simulink model "s_2012"  (Simulink 7.9)
settings: Solver=ode3  SolverMode=SingleTasking  StartTime=0.0  StopTime=10  FixedStep=0.02  MaxStep=0.02  MinStep=0.02  RelTol=1e-3
model workspace: external: MATLAB File I:\mat\ADRC\ass.m (data not in the file)
values from neighbouring files (symbols this model uses):
  a0 = 0.5    [ass.m]    (also in fcn.m = (d^2+8*r*abs(y))^0.5)
  a1 = 0.4    [ass.m]
  a2 = 0.75    [ass.m]
  delta0 = 0.001    [ass.m]
  delta1 = 0.001    [ass.m]
  delta2 = 0.001    [ass.m]
undefined symbols (not defined in the file or in its folder): DiscIntNeverNeededParam
settings Model: Creator=Administrator  LastModifiedBy=Administrator  CovMetricSettings=dwe  CovHtmlReporting=off  covSaveCumulativeToWorkspaceVar=off  CovSaveSingleToWorkspaceVar=off  CovExternalEMLEnable=on
settings SolverCC: InitialStep=0.02
settings DataIOCC: LimitDataPoints=off  SaveFormat=StructureWithTime  SignalLoggingSaveFormat=Dataset  ReturnWorkspaceOutputs=on
settings OptimizationCC: ExpressionDepthLimit=128
settings DebuggingCC: UnderspecifiedInitializationDetection=Simplified  MergeDetectMultiDrivingBlocksExec=error  SolverPrmCheckMsg=none  FrameProcessingCompatibilityMsg=error  StateNameClashWarn=none  SFUnexpectedBacktrackingDiag=error  SFNoUnconditionalDefaultTransitionDiag=error
settings HardwareCC: ProdBitPerPointer=64  ProdLargestAtomicFloat=Float  ProdIntDivRoundTo=Zero  ProdEndianess=LittleEndian  ProdHWDeviceType=Specified
settings ModelReferenceCC: PropagateSignalLabelsOutOfModel=on
settings SFSimCC: SimUseLocalCustomCode=on
settings RTWCC: RTWUseLocalCustomCode=on
settings CodeAppCC: CustomSymbolStrType=$N$R$M_T
settings GRTTargetCC: CodeReplacementLibrary=C99 (ISO)  GeneratePreprocessorConditionals=Use local settings

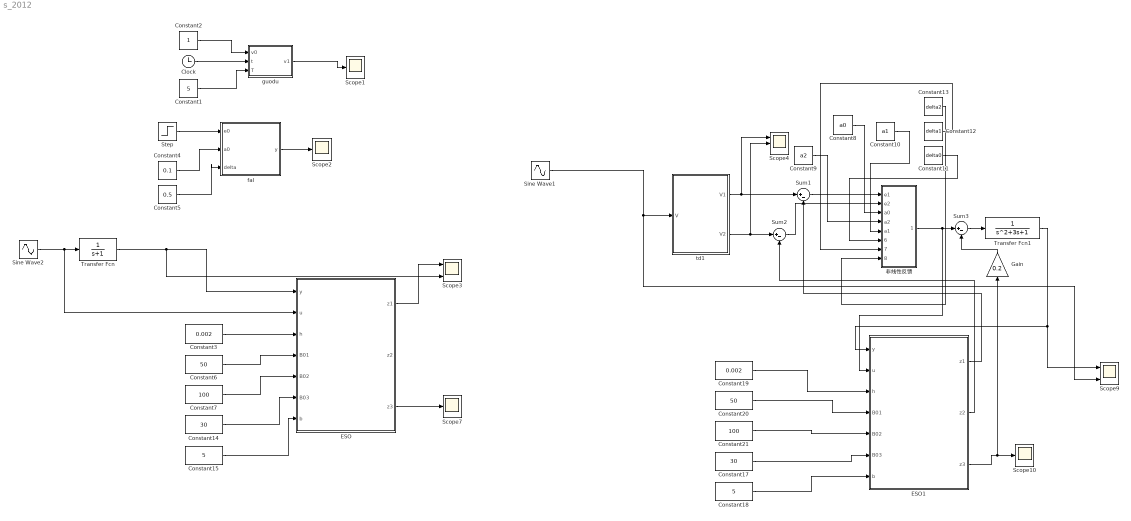
== system s_2012 ==
  Clock : Clock
  Constant1 : Constant  Value=5
  Constant10 : Constant  Value=a1
  Constant11 : Constant  Value=delta0
  Constant12 : Constant  Value=delta1
  Constant13 : Constant  Value=delta2
  Constant14 : Constant  Value=30
  Constant15 : Constant  Value=5
  Constant17 : Constant  Value=30
  Constant18 : Constant  Value=5
  Constant19 : Constant  Value=0.002
  Constant2 : Constant
  Constant20 : Constant  Value=50
  Constant21 : Constant  Value=100
  Constant3 : Constant  Value=0.002
  Constant4 : Constant  Value=0.1
  Constant5 : Constant  Value=0.5
  Constant6 : Constant  Value=50
  Constant7 : Constant  Value=100
  Constant8 : Constant  Value=a0
  Constant9 : Constant  Value=a2
  ESO : Subsystem
  ESO1 : Subsystem
  Gain : Gain  Gain=0.2
  Scope{1..2,7,10} (4 alike) : Scope
      Scope1 settings: TimeRange=auto  MaxDataPoints=5000  SaveToWorkspace=off  YMin=-0.125  YMax=1.125  SampleTime=-1
      Scope10 settings: TimeRange=auto  MaxDataPoints=5000  SaveToWorkspace=off  SaveName=ScopeData3  YMin=-6.92252  YMax=6.95171  SampleTime=-1
      Scope2 settings: TimeRange=auto  MaxDataPoints=5000  SaveToWorkspace=off  SaveName=ScopeData2  YMin=-0.125  YMax=1.125  SampleTime=-1
      Scope7 settings: TimeRange=auto  MaxDataPoints=5000  SaveToWorkspace=off  SaveName=ScopeData8  YMin=-6.95031  YMax=6.9548  SampleTime=-1
  Scope3 : Scope  NumInputPorts=2
      settings: TimeRange=auto  MaxDataPoints=5000  SaveToWorkspace=off  YMin=-0.89002~-5  YMax=0.93911~5  SampleTime=-1
  Scope4 : Scope  NumInputPorts=3
      settings: TimeRange=auto  MaxDataPoints=5000  SaveToWorkspace=off  SaveName=ScopeData3  YMin=-3.68521~-5~-5  YMax=4.43656~5~5  SampleTime=-1
  Scope9 : Scope  NumInputPorts=2
      settings: TimeRange=auto  MaxDataPoints=5000  SaveToWorkspace=off  SaveName=ScopeData4  YMin=-1.45701~-5  YMax=1.50602~5  SampleTime=-1
  Sine Wave1 : Sin  SampleTime=0
  Sine Wave2 : Sin  SampleTime=0
  Step : Step  SampleTime=0
  Sum1 : Sum  Inputs=|+-
  Sum2 : Sum  Inputs=|+-
  Sum3 : Sum  Inputs=|+-
  Transfer Fcn : TransferFcn  Denominator=[1 1]
  Transfer Fcn1 : TransferFcn  Denominator=[1 3 1]
  fal : MATLAB Function  TreatAsAtomicUnit=on
      settings: PermitHierarchicalResolution=ParametersOnly
  guodu : MATLAB Function  TreatAsAtomicUnit=on
      settings: PermitHierarchicalResolution=ParametersOnly
  td1 : Subsystem
  非线性反馈 : Subsystem
  wires:
  Clock/1 -> guodu/2(t)
  Constant1/1 -> guodu/3(T)
  Constant2/1 -> guodu/1(v0)
  guodu/1(v1) -> Scope1/1
  Step/1 -> fal/1(e0)
  Constant4/1 -> fal/2(a0)
  Constant5/1 -> fal/3(delta)
  fal/1(y) -> Scope2/1
  td1/1(V1) -> Scope4/1, Sum1/1
  Sum1/1 -> 非线性反馈/1(e1)
  td1/2(V2) -> Scope4/2, Sum2/1
  Sum2/1 -> 非线性反馈/2(e2)
  Constant10/1 -> 非线性反馈/5(a1)
  Constant9/1 -> 非线性反馈/4(a2)
  Constant8/1 -> 非线性反馈/3(a0)
  Constant11/1 -> 非线性反馈/6(delta0)
  Constant12/1 -> 非线性反馈/7(delta1)
  Constant13/1 -> 非线性反馈/8(delta2)
  Constant3/1 -> ESO/3(h)
  Constant6/1 -> ESO/4(B01)
  Constant7/1 -> ESO/5(B02)
  Constant14/1 -> ESO/6(B03)
  Constant15/1 -> ESO/7(b)
  ESO1/2(z2) -> Sum2/2
  ESO/3(z3) -> Scope7/1
  Sine Wave2/1 -> ESO/2(u), Transfer Fcn/1
  Transfer Fcn/1 -> Scope3/2, ESO/1(y)
  ESO/1(z1) -> Scope3/1
  ESO1/3(z3) -> Gain/1, Scope10/1
  Constant18/1 -> ESO1/7(b)
  Constant17/1 -> ESO1/6(B03)
  Constant21/1 -> ESO1/5(B02)
  Constant19/1 -> ESO1/3(h)
  Constant20/1 -> ESO1/4(B01)
  非线性反馈/1(Out1) -> Sum3/1, ESO1/2(u)
  ESO1/1(z1) -> Sum1/2
  Transfer Fcn1/1 -> ESO1/1(y), Scope9/1
  Sine Wave1/1 -> Scope9/2, td1/1(V)
  Sum3/1 -> Transfer Fcn1/1
  Gain/1 -> Sum3/2

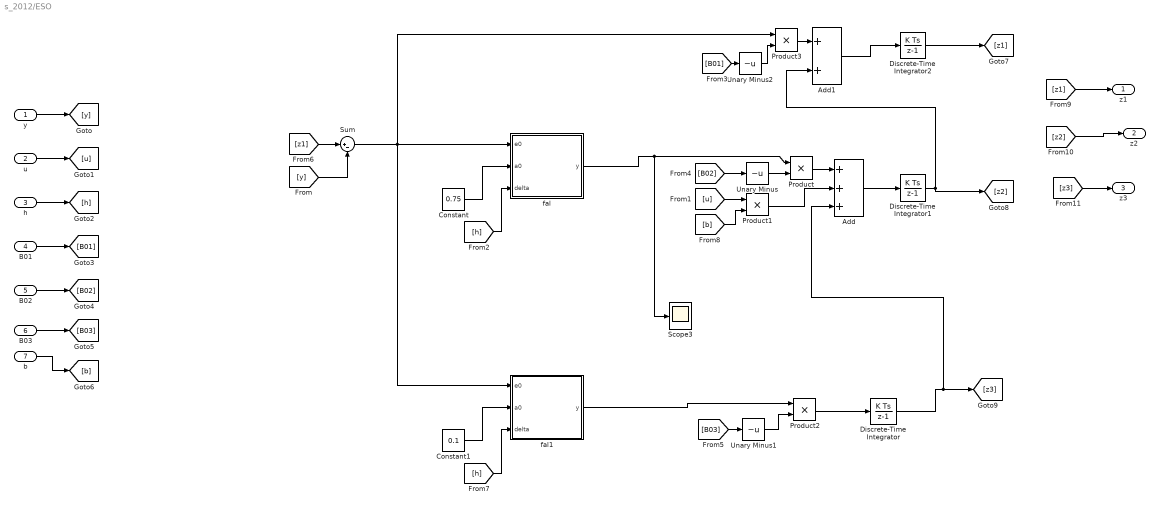
== system s_2012/ESO ==
  y : Inport
  u : Inport  Port=2
  h : Inport  Port=3
  B01 : Inport  Port=4
  B02 : Inport  Port=5
  B03 : Inport  Port=6
  b : Inport  Port=7
  Add : Sum  Inputs=+++
  Add1 : Sum
  Constant : Constant  Value=0.75
  Constant1 : Constant  Value=0.1
  Discrete-Time Integrator : DiscreteIntegrator  InitialConditionMode=State only (most efficient)  SampleTime=-1  ICPrevOutput=DiscIntNeverNeededParam  ICPrevScaledInput=DiscIntNeverNeededParam
  Discrete-Time Integrator1 : DiscreteIntegrator  InitialConditionMode=State only (most efficient)  SampleTime=-1  ICPrevOutput=DiscIntNeverNeededParam  ICPrevScaledInput=DiscIntNeverNeededParam
  Discrete-Time Integrator2 : DiscreteIntegrator  InitialConditionMode=State only (most efficient)  SampleTime=-1  ICPrevOutput=DiscIntNeverNeededParam  ICPrevScaledInput=DiscIntNeverNeededParam
  Product{,1..3} (4 alike) : Product
  Scope3 : Scope
      settings: TimeRange=auto  MaxDataPoints=5000  SaveToWorkspace=off  SaveName=ScopeData2  YMin=-0.00703  YMax=0.01145  SampleTime=-1
  Sum : Sum  Inputs=|+-
  Unary Minus : UnaryMinus
  Unary Minus1 : UnaryMinus
  Unary Minus2 : UnaryMinus
  fal : MATLAB Function  TreatAsAtomicUnit=on
      settings: PermitHierarchicalResolution=ParametersOnly
  fal1 : MATLAB Function  TreatAsAtomicUnit=on
      settings: PermitHierarchicalResolution=ParametersOnly
  z1 : Outport
  z2 : Outport  Port=2
  z3 : Outport  Port=3
  wires:
  y/1 -> [y]
  u/1 -> [u]
  h/1 -> [h]
  B01/1 -> [B01]
  B02/1 -> [B02]
  B03/1 -> [B03]
  [h] -> fal/3(delta)
  [z1] -> Sum/1
  [y] -> Sum/2
  Constant/1 -> fal/2(a0)
  Constant1/1 -> fal1/2(a0)
  [h] -> fal1/3(delta)
  b/1 -> [b]
  [B02] -> Unary Minus/1
  Unary Minus/1 -> Product/2
  [u] -> Product1/1
  [b] -> Product1/2
  Product1/1 -> Add/2
  Product/1 -> Add/1
  fal/1(y) -> Scope3/1, Product/1
  [B03] -> Unary Minus1/1
  Unary Minus1/1 -> Product2/2
  fal1/1(y) -> Product2/1
  [B01] -> Unary Minus2/1
  Sum/1 -> Product3/1, fal1/1(e0), fal/1(e0)
  Unary Minus2/1 -> Product3/2
  Product2/1 -> Discrete-Time Integrator/1
  Add/1 -> Discrete-Time Integrator1/1
  Discrete-Time Integrator2/1 -> [z1]
  Discrete-Time Integrator1/1 -> Add1/2, [z2]
  Discrete-Time Integrator/1 -> Add/3, [z3]
  Product3/1 -> Add1/1
  Add1/1 -> Discrete-Time Integrator2/1
  [z1] -> z1/1
  [z2] -> z2/1
  [z3] -> z3/1

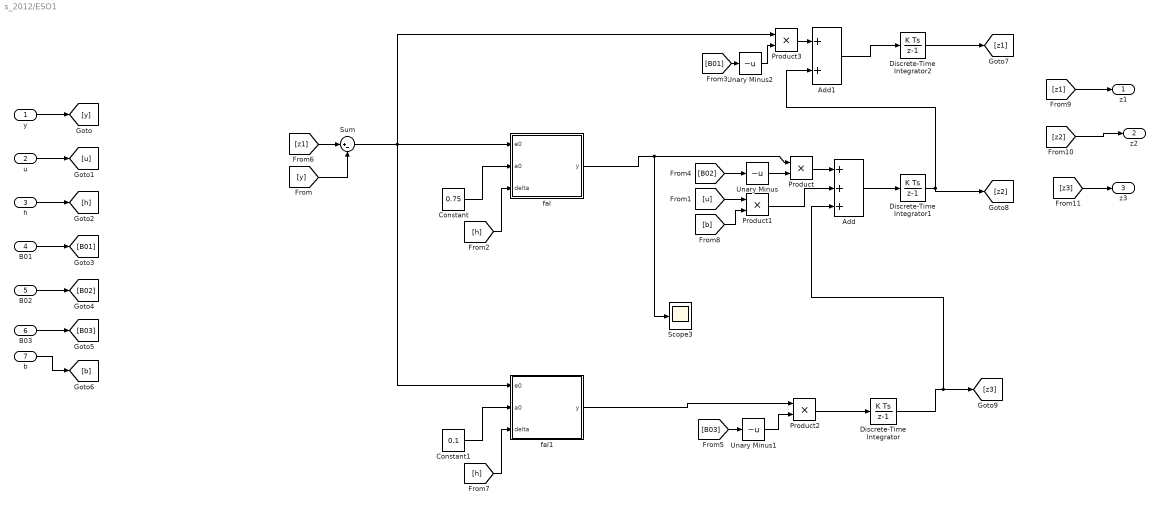
== system s_2012/ESO1 ==
  y : Inport
  u : Inport  Port=2
  h : Inport  Port=3
  B01 : Inport  Port=4
  B02 : Inport  Port=5
  B03 : Inport  Port=6
  b : Inport  Port=7
  Add : Sum  Inputs=+++
  Add1 : Sum
  Constant : Constant  Value=0.75
  Constant1 : Constant  Value=0.1
  Discrete-Time Integrator : DiscreteIntegrator  InitialConditionMode=State only (most efficient)  SampleTime=-1  ICPrevOutput=DiscIntNeverNeededParam  ICPrevScaledInput=DiscIntNeverNeededParam
  Discrete-Time Integrator1 : DiscreteIntegrator  InitialConditionMode=State only (most efficient)  SampleTime=-1  ICPrevOutput=DiscIntNeverNeededParam  ICPrevScaledInput=DiscIntNeverNeededParam
  Discrete-Time Integrator2 : DiscreteIntegrator  InitialConditionMode=State only (most efficient)  SampleTime=-1  ICPrevOutput=DiscIntNeverNeededParam  ICPrevScaledInput=DiscIntNeverNeededParam
  Product{,1..3} (4 alike) : Product
  Scope3 : Scope
      settings: TimeRange=auto  MaxDataPoints=5000  SaveToWorkspace=off  SaveName=ScopeData2  YMin=-0.00703  YMax=0.01145  SampleTime=-1
  Sum : Sum  Inputs=|+-
  Unary Minus : UnaryMinus
  Unary Minus1 : UnaryMinus
  Unary Minus2 : UnaryMinus
  fal : MATLAB Function  TreatAsAtomicUnit=on
      settings: PermitHierarchicalResolution=ParametersOnly
  fal1 : MATLAB Function  TreatAsAtomicUnit=on
      settings: PermitHierarchicalResolution=ParametersOnly
  z1 : Outport
  z2 : Outport  Port=2
  z3 : Outport  Port=3
  wires:
  y/1 -> [y]
  u/1 -> [u]
  h/1 -> [h]
  B01/1 -> [B01]
  B02/1 -> [B02]
  B03/1 -> [B03]
  [h] -> fal/3(delta)
  [z1] -> Sum/1
  [y] -> Sum/2
  Constant/1 -> fal/2(a0)
  Constant1/1 -> fal1/2(a0)
  [h] -> fal1/3(delta)
  b/1 -> [b]
  [B02] -> Unary Minus/1
  Unary Minus/1 -> Product/2
  [u] -> Product1/1
  [b] -> Product1/2
  Product1/1 -> Add/2
  Product/1 -> Add/1
  fal/1(y) -> Scope3/1, Product/1
  [B03] -> Unary Minus1/1
  Unary Minus1/1 -> Product2/2
  fal1/1(y) -> Product2/1
  [B01] -> Unary Minus2/1
  Sum/1 -> Product3/1, fal1/1(e0), fal/1(e0)
  Unary Minus2/1 -> Product3/2
  Product2/1 -> Discrete-Time Integrator/1
  Add/1 -> Discrete-Time Integrator1/1
  Discrete-Time Integrator2/1 -> [z1]
  Discrete-Time Integrator1/1 -> Add1/2, [z2]
  Discrete-Time Integrator/1 -> Add/3, [z3]
  Product3/1 -> Add1/1
  Add1/1 -> Discrete-Time Integrator2/1
  [z1] -> z1/1
  [z2] -> z2/1
  [z3] -> z3/1

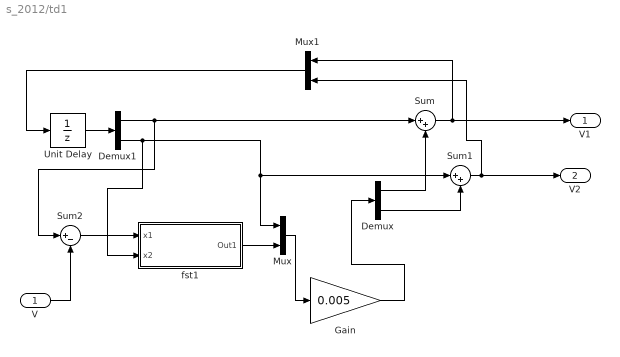
== system s_2012/td1 ==
  V : Inport
  Demux : Demux  Outputs=2
  Demux1 : Demux  Outputs=2
  Gain : Gain  Gain=0.005
  Mux : Mux  Inputs=2
  Mux1 : Mux  Inputs=2
  Sum : Sum  Inputs=|++
  Sum1 : Sum  Inputs=|++
  Sum2 : Sum  Inputs=|+-
  Unit Delay : UnitDelay  SampleTime=-1  HasFrameUpgradeWarning=on
  fst1 : Subsystem
  V1 : Outport
  V2 : Outport  Port=2
  wires:
  Mux/1 -> Gain/1
  fst1/1(Out1) -> Mux/2
  Gain/1 -> Demux/1
  Demux/1 -> Sum/2
  Demux/2 -> Sum1/2
  Sum1/1 -> V2/1, Mux1/2
  Sum/1 -> V1/1, Mux1/1
  Unit Delay/1 -> Demux1/1
  Mux1/1 -> Unit Delay/1
  V/1 -> Sum2/2
  Sum2/1 -> fst1/1(x1)
  Demux1/1 -> Sum2/1, Sum/1
  Demux1/2 -> fst1/2(x2), Mux/1, Sum1/1

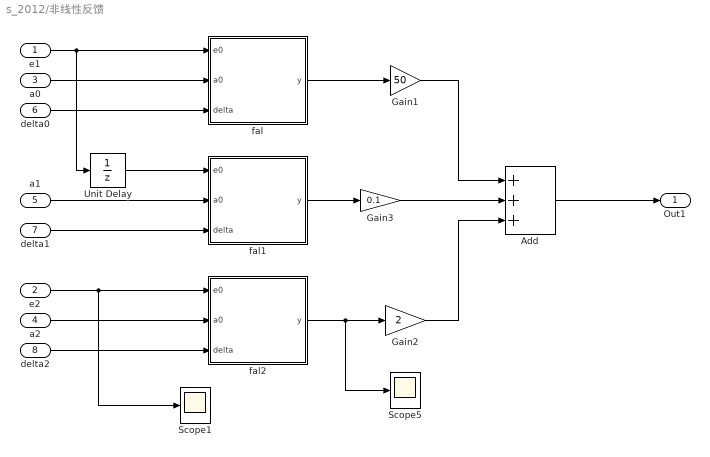
== system s_2012/非线性反馈 ==
  e1 : Inport
  e2 : Inport  Port=2
  a0 : Inport  Port=3
  a2 : Inport  Port=4
  a1 : Inport  Port=5
  delta0 : Inport  Port=6
  delta1 : Inport  Port=7
  delta2 : Inport  Port=8
  Add : Sum  Inputs=+++
  Gain1 : Gain  Gain=50
  Gain2 : Gain  Gain=2
  Gain3 : Gain  Gain=0.1
  Scope1 : Scope
      settings: TimeRange=auto  MaxDataPoints=5000  SaveToWorkspace=off  SaveName=ScopeData6  YMin=-4.98591  YMax=4.99422  SampleTime=-1
  Scope5 : Scope
      settings: TimeRange=auto  MaxDataPoints=5000  SaveToWorkspace=off  SaveName=ScopeData5  YMin=-3.52806  YMax=3.53247  SampleTime=-1
  Unit Delay : UnitDelay  SampleTime=-1  HasFrameUpgradeWarning=on
  fal : MATLAB Function  TreatAsAtomicUnit=on
      settings: PermitHierarchicalResolution=ParametersOnly
  fal1 : MATLAB Function  TreatAsAtomicUnit=on
      settings: PermitHierarchicalResolution=ParametersOnly
  fal2 : MATLAB Function  TreatAsAtomicUnit=on
      settings: PermitHierarchicalResolution=ParametersOnly
  Out1 : Outport
  wires:
  e1/1 -> Unit Delay/1, fal/1(e0)
  e2/1 -> Scope1/1, fal2/1(e0)
  Unit Delay/1 -> fal1/1(e0)
  a0/1 -> fal/2(a0)
  a2/1 -> fal2/2(a0)
  a1/1 -> fal1/2(a0)
  delta0/1 -> fal/3(delta)
  delta1/1 -> fal1/3(delta)
  delta2/1 -> fal2/3(delta)
  fal1/1(y) -> Gain3/1
  fal/1(y) -> Gain1/1
  fal2/1(y) -> Gain2/1, Scope5/1
  Gain1/1 -> Add/1
  Gain2/1 -> Add/3
  Gain3/1 -> Add/2
  Add/1 -> Out1/1

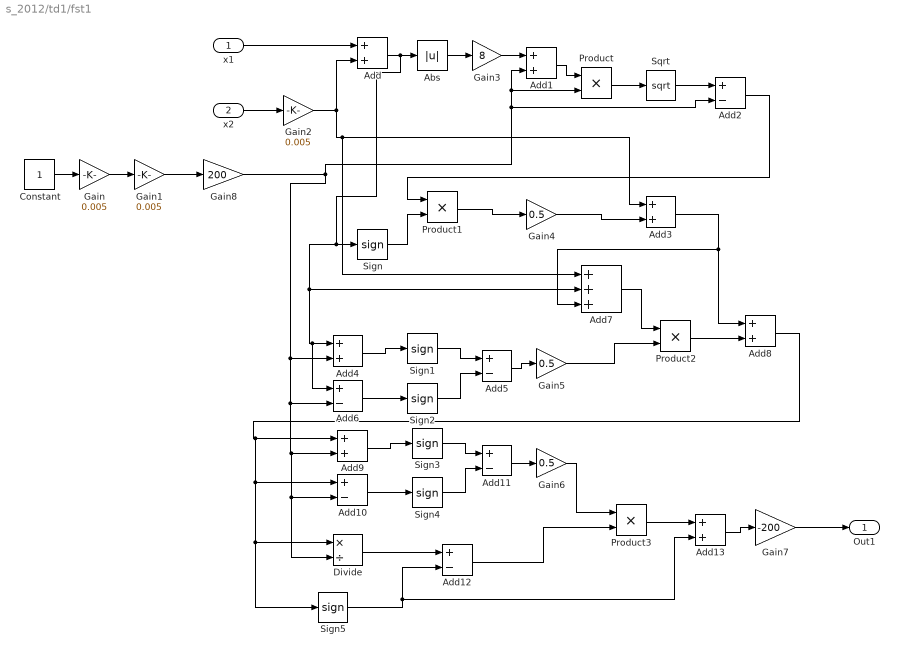
== system s_2012/td1/fst1 ==
  x1 : Inport
  x2 : Inport  Port=2
  Abs : Abs
  Add{,1,3..4,8..9,13} (7 alike) : Sum
  Add{2,5..6,10..12} (6 alike) : Sum  Inputs=+-
  Add7 : Sum  Inputs=+++
  Constant : Constant
  Divide : Product  Inputs=*/
  Gain : Gain  Gain=0.005
  Gain1 : Gain  Gain=0.005
  Gain2 : Gain  Gain=0.005
  Gain3 : Gain  Gain=8
  Gain4 : Gain  Gain=0.5
  Gain5 : Gain  Gain=0.5
  Gain6 : Gain  Gain=0.5
  Gain7 : Gain  Gain=-200
  Gain8 : Gain  Gain=200
  Product{,1..3} (4 alike) : Product
  Sign{,1..5} (6 alike) : Signum
  Sqrt : Sqrt  SaturateOnIntegerOverflow=on
  Out1 : Outport
  wires:
  Constant/1 -> Gain/1
  Gain/1 -> Gain1/1
  x2/1 -> Gain2/1
  x1/1 -> Add/1
  Gain2/1 -> Add7/1, Add3/1, Add/2
  Add/1 -> Add6/1, Add4/1, Add7/2, Sign/1, Abs/1
  Abs/1 -> Gain3/1
  Gain3/1 -> Add1/1
  Add1/1 -> Product/1
  Product/1 -> Sqrt/1
  Sqrt/1 -> Add2/1
  Gain1/1 -> Gain8/1
  Sign/1 -> Product1/2
  Add2/1 -> Product1/1
  Product1/1 -> Gain4/1
  Gain4/1 -> Add3/2
  Add4/1 -> Sign1/1
  Sign1/1 -> Add5/1
  Add6/1 -> Sign2/1
  Sign2/1 -> Add5/2
  Add5/1 -> Gain5/1
  Add7/1 -> Product2/1
  Gain5/1 -> Product2/2
  Add3/1 -> Add7/3, Add8/1
  Product2/1 -> Add8/2
  Add10/1 -> Sign4/1
  Add9/1 -> Sign3/1
  Sign4/1 -> Add11/2
  Sign3/1 -> Add11/1
  Add8/1 -> Sign5/1, Divide/1, Add10/1, Add9/1
  Add11/1 -> Gain6/1
  Divide/1 -> Add12/1
  Sign5/1 -> Add13/2, Add12/2
  Gain6/1 -> Product3/1
  Add12/1 -> Product3/2
  Product3/1 -> Add13/1
  Add13/1 -> Gain7/1
  Gain7/1 -> Out1/1
  Gain8/1 -> Add2/2, Product/2, Add1/2, Divide/2, Add10/2, Add9/2, Add6/2, Add4/2

== matlab function guodu ==
  data: v0 input double; v1 output double; t input double; T input double
function v1 = fcn(v0,t,T)

if(t<=(T/2))
 v1=2*v0/(T^2)*(t^2);
elseif(t<=T)
    v1=v0*(-2*t^2/(T^2)+4*t/T-1);
else
    v1=v0;
end

== matlab function fal ==
  data: e0 input double; y output double; a0 input double; delta input double
function y = fcn(e0,a0,delta)
if(abs(e0)>delta)
    y=(abs(e0))^a0*sign(e0);
else
    y=e0/(delta^(1-a0));
end

== matlab function ESO/fal ==
  data: e0 input double; y output double; a0 input double; delta input double
function y = fcn(e0,a0,delta)
if(abs(e0)>delta)
    y=((abs(e0))^a0)*sign(e0);
else
    y=e0/(delta^(1-a0));
end

== matlab function ESO/fal1 ==
  data: e0 input double; y output double; a0 input double; delta input double
function y = fcn(e0,a0,delta)
if(abs(e0)>delta)
    y=(abs(e0))^a0*sign(e0);
else
    y=e0/(delta^(1-a0));
end

== matlab function 非线性反馈/fal ==
  data: e0 input double; y output double; a0 input double; delta input double
function y = fcn(e0,a0,delta)
if(abs(e0)>delta)
    y=(abs(e0))^a0*sign(e0);
else
    y=e0/(delta^(1-a0));
end

== matlab function 非线性反馈/fal1 ==
  data: e0 input double; y output double; a0 input double; delta input double
function y = fcn(e0,a0,delta)
if(abs(e0)>delta)
    y=(abs(e0))^a0*sign(e0);
else
    y=e0/(delta^(1-a0));
end

== matlab function 非线性反馈/fal2 ==
  data: e0 input double; y output double; a0 input double; delta input double
function y = fcn(e0,a0,delta)
if(abs(e0)>delta)
    y=(abs(e0))^a0*sign(e0);
else
    y=e0/(delta^(1-a0));
end

== matlab function ESO1/fal ==
  data: e0 input double; y output double; a0 input double; delta input double
function y = fcn(e0,a0,delta)
if(abs(e0)>delta)
    y=((abs(e0))^a0)*sign(e0);
else
    y=e0/(delta^(1-a0));
end

== matlab function ESO1/fal1 ==
  data: e0 input double; y output double; a0 input double; delta input double
function y = fcn(e0,a0,delta)
if(abs(e0)>delta)
    y=(abs(e0))^a0*sign(e0);
else
    y=e0/(delta^(1-a0));
end
